simulink model "UAV_SIL"  (Simulink 8.4)
settings: Solver=ode3  StartTime=0.0  StopTime=40  FixedStep=SampleTime  RelTol=1e-3
values from neighbouring files (symbols this model uses):
  IntegerTimeDelay = 2    [setup.m]
undefined symbols (not defined in the file or in its folder): OperatingPoint, TrimCondition
undefined symbols (not defined in the file): AC
libraries: Actuator_Lib x2, Environment_Lib x1, simulink x1, NonlinearModel_Lib x1, Sensors_Lib x1
settings Model: Creator=Paul Freeman  LastModifiedBy=PC
settings DataIOCC: LimitDataPoints=off  SaveOutput=off  SignalLogging=off
settings HardwareCC: ProdLargestAtomicInteger=Long  ProdLargestAtomicFloat=Double  ProdIntDivRoundTo=Zero  ProdEndianess=BigEndian  ProdHWDeviceType=Freescale->32-bit PowerPC
settings SFSimCC: SimParseCustomCode=off

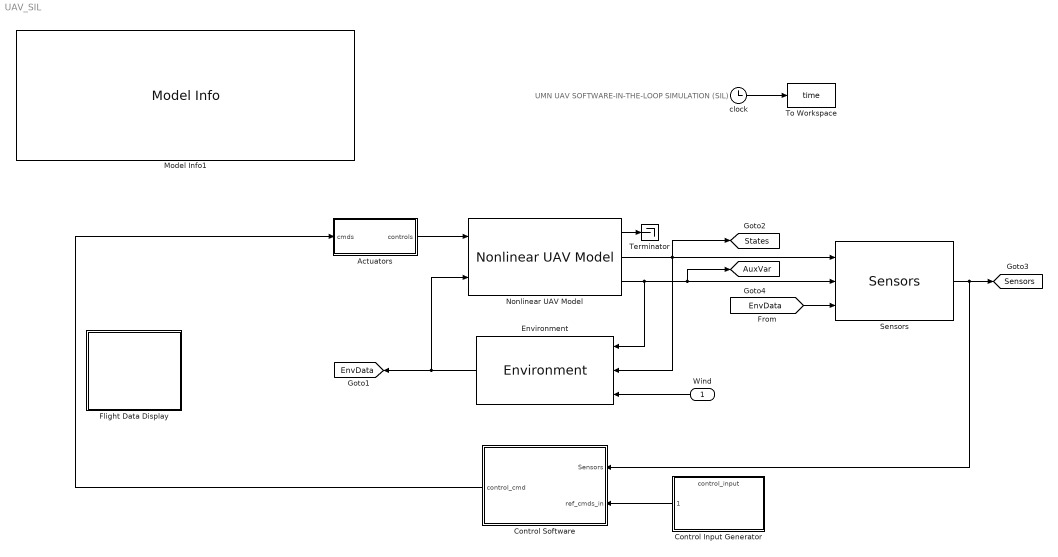
== system UAV_SIL ==
  note: UMN UAV
      | SOFTWARE-IN-THE-LOOP SIMULATION
      | (SIL)
  Wind : Inport  PortDimensions=3
  Actuators : Subsystem  BlockChoice=miniMUTT  mask{aircraft=AC.aircraft}
      mask help: Set actuator models, either 'UltraStick120', 'UltraStick25e', or 'miniMUTT'
      mask init:
      | pathname = gcb;
      | 
      | switch lower(aircraft)
      |     case 'ultrastick120'
      |         set_param(pathname,'BlockChoice','UltraStick');
      |     case 'ultrastick25e'
      |         set_param(pathname,'BlockChoice','UltraStick');
      |     case 'minimutt'
      |         set_param(pathname,'BlockChoice','miniMUTT');
      |     case 'rigid_minimutt'
      |         set_param(pathname,'BlockChoice','miniMUTT');
      | end
      settings: AttributesFormatString=%<BlockChoice>  TemplateBlock=Actuator_Lib/Actuators  MemberBlocks=UltraStick,miniMUTT
  Control Input Generator : ModelReference  ModelNameDialog=control_input  SimulationMode=Normal  ModelReferenceVersion=1.90  CopyOfModelName=control_input  DefaultDataLogging=off
  Control Software : Subsystem
  Environment : Environment_Lib/Environment
  Flight Data Display : Subsystem
      mask Display:
      | x = 0:.1:2*pi;
      | plot(x,sin(x)+rand(size(x))*.5)
  Model Info1 : simulink/Model-Wide Utilities/Model Info  BlockCM=None  Frame=on  DisplayStringWithTags=|  HorizontalTextAlignment=Left  LeftAlignmentValue=0.02  SourceBlockDiagram=UAV_SIL  TagMaxNumber=20
      | MODEL INFORMATION
      | UMN UAV Software-in-the-Loop Simulation
      | 
      | University of Minnesota
      | Aerospace Engineering and Mechanics
      | Copyright 2011 Regents of the University of Minnesota. All rights reserved.
      | 
      | == SVN Info ==
      | Last modified by %<LastModifiedBy> on %<LastModificationDate>
  Nonlinear UAV Model : NonlinearModel_Lib/Nonlinear UAV Model
      link override Forces and Moments/Electric Propulsion Forces and Moments: BlockChoice=miniMUTT
  Sensors : Sensors_Lib/Sensors
  Terminator : Terminator
  To Workspace : ToWorkspace  VariableName=time  SampleTime=-1
  clock : Clock
  tag scope: AuxVar=global, EnvData=global, Sensors=global, States=global
  wires:
  Sensors/1 -> Control Software/1(Sensors), [Sensors]
  Control Software/1(control_cmd) -> Actuators/1(cmds)
  Actuators/1(controls) -> Nonlinear UAV Model/1
  clock/1 -> To Workspace/1
  Control Input Generator/1 -> Control Software/2(ref_cmds_in)
  Nonlinear UAV Model/1 -> Terminator/1
  Environment/1 -> [EnvData], Nonlinear UAV Model/2
  Nonlinear UAV Model/3 -> Environment/1, [AuxVar], Sensors/2
  Nonlinear UAV Model/2 -> Environment/2, Sensors/1, [States]
  [EnvData] -> Sensors/3
  Wind/1 -> Environment/3

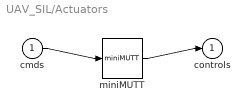
== system UAV_SIL/Actuators ==
  cmds : Inport
  miniMUTT : Actuator_Lib/miniMUTT
  controls : Outport
  wires:
  cmds/1 -> miniMUTT/1
  miniMUTT/1 -> controls/1

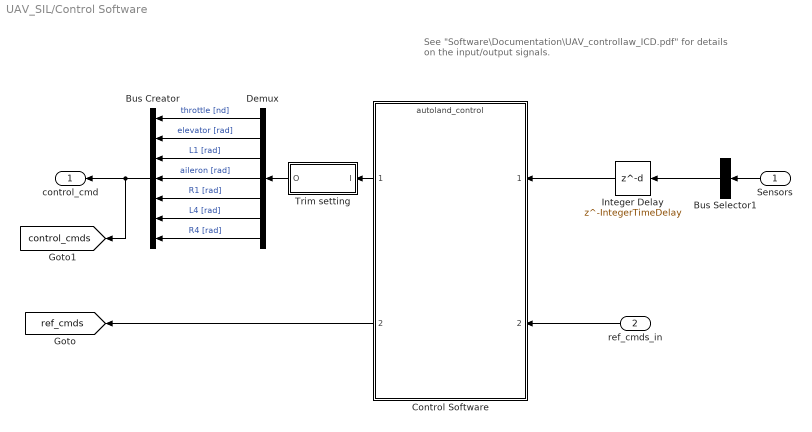
== system UAV_SIL/Control Software ==
  note: See "Software\Documentation\UAV_controllaw_ICD.pdf" for
      | details on the input/output signals.
  Sensors : Inport
  ref_cmds_in : Inport  Port=2
  Bus Creator : BusCreator  Inputs=7
  Bus Selector1 : BusSelector  OutputSignals=phi [rad],theta [rad],psi [rad],p [rad/s],q [rad/s],r [rad/s],Ax [m/s^2],Ay [m/s^2],Az [m/s^2],h [m],V_s [m/s],alpha [rad],beta [rad],Geodetic Latitude [rad],Geodetic Longitude [rad],Altitude [m],Xdot [m/s],Ydot [m/s],Zdot [m/s]  OutputAsBus=on
  Control Software : ModelReference  ModelNameDialog=autoland_control  Variant=on  ModelReferenceVersion=1.224  CopyOfModelName=autoland_control  DefaultDataLogging=off
  Demux : Demux  Outputs=7
  Integer Delay : Delay  DelayLength=IntegerTimeDelay  InitialCondition=repmat([TrimCondition.AttitudeIni;TrimCondition.RatesIni;TrimCondition.AccelsIni;OperatingPoint.op_report.Outputs(4).y;TrimCondition.WindAxesIni;TrimCondition.LLIni;0; zeros(3,1)],[1,IntegerTimeDelay])  InputProcessing=Inherited
  Trim setting : Subsystem  BlockChoice=Trim setting MiniMUTT  mask{aircraft=AC.aircraft}
      link override Trim setting MiniMUTT/Control Surfaces trim: Value=[TrimCondition.Inputs.CtrlSurf(1) TrimCondition.Inputs.CtrlSurf(2) TrimCondition.Inputs.CtrlSurf(3) TrimCondition.Inputs.CtrlSurf(4) TrimCondition.Inputs.CtrlSurf(5) TrimCondition.Inputs.CtrlSurf(6)]
      link override Trim setting MiniMUTT/Throttle trim: Value=TrimCondition.Inputs.Throttle
      mask prompts: aircraft "Aircraft model"
      mask init:
      | pathname = gcb;
      | 
      | switch lower(aircraft)
      |     case 'ultrastick120'
      |         set_param(pathname,'BlockChoice','Trim setting UltraStick');
      |     case 'ultrastick25e'
      |         set_param(pathname,'BlockChoice','Trim setting UltraStick');
      |     case 'minimutt'
      |         set_param(pathname,'BlockChoice','Trim setting MiniMUTT');
      |     case 'rigid_minimutt'
      |         set_param(pathname,'BlockChoice','Trim setting MiniMUTT');
      | end
      settings: AttributesFormatString=%<BlockChoice>  TemplateBlock=Actuator_Lib/Trim setting  MemberBlocks=Trim setting MiniMUTT,Trim setting UltraStick
  control_cmd : Outport
  tag scope: control_cmds=global, ref_cmds=global
  wires:
  Sensors/1 -> Bus Selector1/1
  ref_cmds_in/1 -> Control Software/2
  Bus Creator/1 -> control_cmd/1, [control_cmds]
  Demux/1 -> Bus Creator/1  "throttle [nd]"
  Demux/2 -> Bus Creator/2  "elevator [rad]"
  Demux/3 -> Bus Creator/3  "L1 [rad]"
  Demux/4 -> Bus Creator/4  "aileron [rad]"
  Demux/5 -> Bus Creator/5  "R1 [rad]"
  Demux/6 -> Bus Creator/6  "L4 [rad]"
  Demux/7 -> Bus Creator/7  "R4 [rad]"
  Integer Delay/1 -> Control Software/1
  Bus Selector1/1 -> Integer Delay/1
  Control Software/2 -> [ref_cmds]
  Trim setting/1(O) -> Demux/1
  Control Software/1 -> Trim setting/1(I)

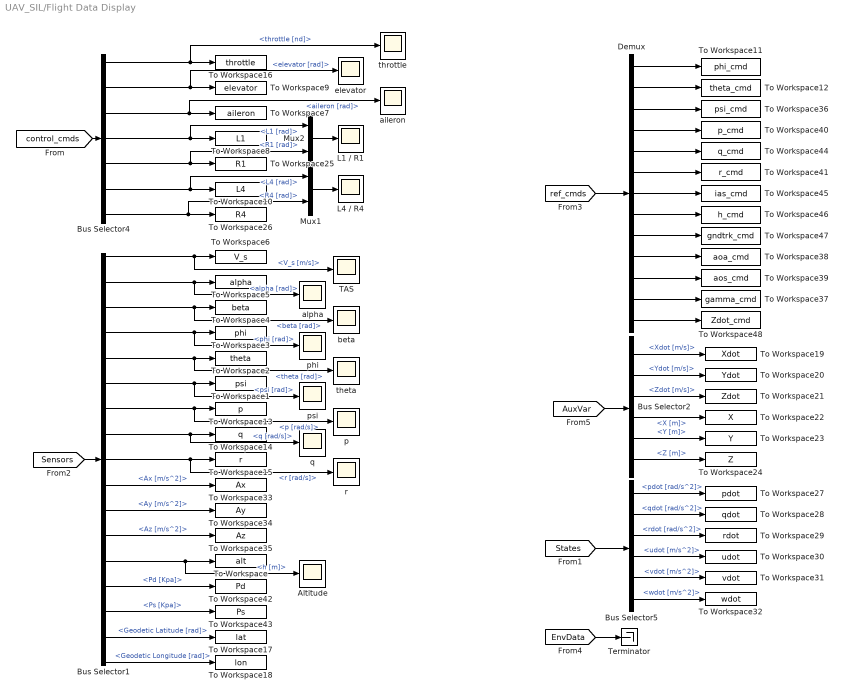
== system UAV_SIL/Flight Data Display ==
  Altitude : Scope
      settings: TimeRange=60  YMin=75  YMax=115  SaveName=ScopeData10
  Bus Selector1 : BusSelector  OutputSignals=V_s [m/s],alpha [rad],beta [rad],phi [rad],theta [rad],psi [rad],p [rad/s],q [rad/s],r [rad/s],Ax [m/s^2],Ay [m/s^2],Az [m/s^2],h [m],Pd [Kpa],Ps [Kpa],Geodetic Latitude [rad],Geodetic Longitude [rad]
  Bus Selector2 : BusSelector  OutputSignals=V_e [m/s].Xdot [m/s],V_e [m/s].Ydot [m/s],V_e [m/s].Zdot [m/s],X_e [m].X [m],X_e [m].Y [m],X_e [m].Z [m]
  Bus Selector4 : BusSelector  OutputSignals=throttle [nd],elevator [rad],aileron [rad],L1 [rad],R1 [rad],L4 [rad],R4 [rad]
  Bus Selector5 : BusSelector  OutputSignals=AngAccel [rad/s^2].pdot [rad/s^2],AngAccel [rad/s^2].qdot [rad/s^2],AngAccel [rad/s^2].rdot [rad/s^2],A_b [m/s^2].udot [m/s^2],A_b [m/s^2].vdot [m/s^2],A_b [m/s^2].wdot [m/s^2]
  Demux : Demux  Outputs=13
  L1 / R1 : Scope
      settings: TimeRange=20  YMin=-20  YMax=20  SaveName=ScopeData2
  L4 / R4 : Scope
      settings: TimeRange=20  YMin=-20  YMax=20  SaveName=ScopeData5
  Mux1 : Mux  Inputs=2
  Mux2 : Mux  Inputs=2
  TAS : Scope
      settings: TimeRange=45  YMin=14  YMax=19  SaveName=ScopeData3
  Terminator : Terminator
  To Workspace : ToWorkspace  VariableName=alt  SampleTime=-1
  To Workspace1 : ToWorkspace  VariableName=psi  SampleTime=-1
  To Workspace10 : ToWorkspace  VariableName=L4  SampleTime=-1
  To Workspace11 : ToWorkspace  VariableName=phi_cmd  SampleTime=-1
  To Workspace12 : ToWorkspace  VariableName=theta_cmd  SampleTime=-1
  To Workspace13 : ToWorkspace  VariableName=p  SampleTime=-1
  To Workspace14 : ToWorkspace  VariableName=q  SampleTime=-1
  To Workspace15 : ToWorkspace  VariableName=r  SampleTime=-1
  To Workspace16 : ToWorkspace  VariableName=throttle  SampleTime=-1
  To Workspace17 : ToWorkspace  VariableName=lat  SampleTime=-1
  To Workspace18 : ToWorkspace  VariableName=lon  SampleTime=-1
  To Workspace19 : ToWorkspace  VariableName=Xdot  SampleTime=-1
  To Workspace2 : ToWorkspace  VariableName=theta  SampleTime=-1
  To Workspace20 : ToWorkspace  VariableName=Ydot  SampleTime=-1
  To Workspace21 : ToWorkspace  VariableName=Zdot  SampleTime=-1
  To Workspace22 : ToWorkspace  VariableName=X  SampleTime=-1
  To Workspace23 : ToWorkspace  VariableName=Y  SampleTime=-1
  To Workspace24 : ToWorkspace  VariableName=Z  SampleTime=-1
  To Workspace25 : ToWorkspace  VariableName=R1  SampleTime=-1
  To Workspace26 : ToWorkspace  VariableName=R4  SampleTime=-1
  To Workspace27 : ToWorkspace  VariableName=pdot  SampleTime=-1
  To Workspace28 : ToWorkspace  VariableName=qdot  SampleTime=-1
  To Workspace29 : ToWorkspace  VariableName=rdot  SampleTime=-1
  To Workspace3 : ToWorkspace  VariableName=phi  SampleTime=-1
  To Workspace30 : ToWorkspace  VariableName=udot  SampleTime=-1
  To Workspace31 : ToWorkspace  VariableName=vdot  SampleTime=-1
  To Workspace32 : ToWorkspace  VariableName=wdot  SampleTime=-1
  To Workspace33 : ToWorkspace  VariableName=Ax  SampleTime=-1
  To Workspace34 : ToWorkspace  VariableName=Ay  SampleTime=-1
  To Workspace35 : ToWorkspace  VariableName=Az  SampleTime=-1
  To Workspace36 : ToWorkspace  VariableName=psi_cmd  SampleTime=-1
  To Workspace37 : ToWorkspace  VariableName=gamma_cmd  SampleTime=-1
  To Workspace38 : ToWorkspace  VariableName=aoa_cmd  SampleTime=-1
  To Workspace39 : ToWorkspace  VariableName=aos_cmd  SampleTime=-1
  To Workspace4 : ToWorkspace  VariableName=beta  SampleTime=-1
  To Workspace40 : ToWorkspace  VariableName=p_cmd  SampleTime=-1
  To Workspace41 : ToWorkspace  VariableName=r_cmd  SampleTime=-1
  To Workspace42 : ToWorkspace  VariableName=Pd  SampleTime=-1
  To Workspace43 : ToWorkspace  VariableName=Ps  SampleTime=-1
  To Workspace44 : ToWorkspace  VariableName=q_cmd  SampleTime=-1
  To Workspace45 : ToWorkspace  VariableName=ias_cmd  SampleTime=-1
  To Workspace46 : ToWorkspace  VariableName=h_cmd  SampleTime=-1
  To Workspace47 : ToWorkspace  VariableName=gndtrk_cmd  SampleTime=-1
  To Workspace48 : ToWorkspace  VariableName=Zdot_cmd  SampleTime=-1
  To Workspace5 : ToWorkspace  VariableName=alpha  SampleTime=-1
  To Workspace6 : ToWorkspace  VariableName=V_s  SampleTime=-1
  To Workspace7 : ToWorkspace  VariableName=aileron  SampleTime=-1
  To Workspace8 : ToWorkspace  VariableName=L1  SampleTime=-1
  To Workspace9 : ToWorkspace  VariableName=elevator  SampleTime=-1
  aileron : Scope
      settings: TimeRange=45  YMin=-1.5  YMax=2  SaveName=ScopeData4
  alpha : Scope
      settings: TimeRange=25  YMin=0.035  YMax=0.08  SaveName=ScopeData7
  beta : Scope
      settings: TimeRange=25  YMin=-0.06  YMax=0.06  SaveName=ScopeData11
  elevator : Scope
      settings: TimeRange=45  YMin=4  YMax=6.5
  p : Scope
      settings: TimeRange=45  YMin=-60  YMax=30  SaveName=ScopeData8
  phi : Scope
      settings: TimeRange=20  YMin=-25  YMax=25  SaveName=ScopeData14
  psi : Scope
      settings: TimeRange=20  YMin=0  YMax=375  SaveName=ScopeData12
  q : Scope
      settings: TimeRange=45  YMax=4  SaveName=ScopeData9
  r : Scope
      settings: TimeRange=45  YMin=-8  YMax=8
  theta : Scope
      settings: TimeRange=20  YMin=0  YMax=3.25  SaveName=ScopeData13
  throttle : Scope
      settings: TimeRange=25  YMin=0.4  YMax=0.75  SaveName=ScopeData15
  wires:
  [States] -> Bus Selector5/1
  Bus Selector4/1 -> To Workspace16/1, throttle/1  "<throttle [nd]>"
  Bus Selector4/2 -> To Workspace9/1, elevator/1  "<elevator [rad]>"
  Bus Selector4/4 -> Mux2/1, To Workspace8/1  "<L1 [rad]>"
  Bus Selector4/5 -> To Workspace25/1, Mux2/2  "<R1 [rad]>"
  Mux2/1 -> L1 / R1/1
  [control_cmds] -> Bus Selector4/1
  [Sensors] -> Bus Selector1/1
  Bus Selector1/7 -> To Workspace13/1, p/1  "<p [rad/s]>"
  Bus Selector1/8 -> To Workspace14/1, q/1  "<q [rad/s]>"
  Bus Selector1/9 -> To Workspace15/1, r/1  "<r [rad/s]>"
  Bus Selector1/10 -> To Workspace33/1  "<Ax [m/s^2]>"
  Bus Selector1/11 -> To Workspace34/1  "<Ay [m/s^2]>"
  Bus Selector1/12 -> To Workspace35/1  "<Az [m/s^2]>"
  Bus Selector1/13 -> To Workspace/1, Altitude/1  "<h [m]>"
  Bus Selector1/14 -> To Workspace42/1  "<Pd [Kpa]>"
  Bus Selector1/15 -> To Workspace43/1  "<Ps [Kpa]>"
  Bus Selector1/16 -> To Workspace17/1  "<Geodetic Latitude [rad]>"
  Bus Selector1/17 -> To Workspace18/1  "<Geodetic Longitude [rad]>"
  [EnvData] -> Terminator/1
  Bus Selector1/6 -> To Workspace1/1, psi/1  "<psi [rad]>"
  Bus Selector1/1 -> To Workspace6/1, TAS/1  "<V_s [m/s]>"
  Bus Selector1/2 -> To Workspace5/1, alpha/1  "<alpha [rad]>"
  Bus Selector1/3 -> To Workspace4/1, beta/1  "<beta [rad]>"
  Bus Selector1/4 -> To Workspace3/1, phi/1  "<phi [rad]>"
  Bus Selector1/5 -> To Workspace2/1, theta/1  "<theta [rad]>"
  [ref_cmds] -> Demux/1
  Demux/1 -> To Workspace11/1
  Demux/2 -> To Workspace12/1
  Demux/3 -> To Workspace36/1
  Demux/4 -> To Workspace40/1
  Demux/5 -> To Workspace44/1
  Demux/6 -> To Workspace41/1
  Demux/7 -> To Workspace45/1
  Demux/8 -> To Workspace46/1
  Demux/9 -> To Workspace47/1
  Demux/10 -> To Workspace38/1
  Demux/11 -> To Workspace39/1
  Demux/12 -> To Workspace37/1
  Bus Selector5/1 -> To Workspace27/1  "<pdot [rad/s^2]>"
  Bus Selector5/2 -> To Workspace28/1  "<qdot [rad/s^2]>"
  Bus Selector5/3 -> To Workspace29/1  "<rdot [rad/s^2]>"
  Bus Selector5/4 -> To Workspace30/1  "<udot [m/s^2]>"
  Bus Selector5/5 -> To Workspace31/1  "<vdot [m/s^2]>"
  Bus Selector5/6 -> To Workspace32/1  "<wdot [m/s^2]>"
  [AuxVar] -> Bus Selector2/1
  Bus Selector2/1 -> To Workspace19/1  "<Xdot [m/s]>"
  Bus Selector2/2 -> To Workspace20/1  "<Ydot [m/s]>"
  Bus Selector2/3 -> To Workspace21/1  "<Zdot [m/s]>"
  Bus Selector2/4 -> To Workspace22/1  "<X [m]>"
  Bus Selector2/5 -> To Workspace23/1  "<Y [m]>"
  Bus Selector2/6 -> To Workspace24/1  "<Z [m]>"
  Bus Selector4/6 -> Mux1/1, To Workspace10/1  "<L4 [rad]>"
  Bus Selector4/7 -> Mux1/2, To Workspace26/1  "<R4 [rad]>"
  Mux1/1 -> L4 / R4/1
  Bus Selector4/3 -> aileron/1, To Workspace7/1  "<aileron [rad]>"
  Demux/13 -> To Workspace48/1

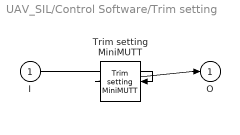
== system UAV_SIL/Control Software/Trim setting ==
  I : Inport
  Trim setting MiniMUTT : Actuator_Lib/Trim setting MiniMUTT
  O : Outport
  wires:
  I/1 -> Trim setting MiniMUTT/1
  Trim setting MiniMUTT/1 -> O/1
